simulink model "ORMComponent"  (R2024a)
settings: Solver=FixedStepAuto  StartTime=0.0  StopTime=10.0  RelTol=1e-3
settings Model: DataDictionary=untitled_dict1.sldd  Creator=diell  LastModifiedBy=diell
settings OptimizationCC: DefaultParameterBehavior=Inlined  EnhancedBackFolding=on  PassReuseOutputArgsAs=Individual arguments  ZeroExternalMemoryAtStartup=off  ZeroInternalMemoryAtStartup=off  OptimizeBlockOrder=speed  DifferentSizesBufferReuse=on  OptimizationCustomize=off  EfficientTunableParamExpr=on
settings DebuggingCC: ParameterTunabilityLossMsg=error
settings SFSimCC: MATLABDynamicMemAlloc=off
settings RTWCC: Description=Embedded Coder  SystemTargetFile=ert.tlc  TemplateMakefile=ert_default_tmf  TargetLang=C++
settings CodeAppCC: ForceParamTrailComments=on  IgnoreCustomStorageClasses=off  OperatorAnnotations=on  SimulinkDataObjDesc=on  SFDataObjDesc=on  InsertBlockDesc=on
settings ERTTargetCC: TargetLangStandard=C++11 (ISO)  GenerateSampleERTMain=on  CodeInterfacePackaging=C++ class  InlinedParameterPlacement=NonHierarchical  RootIOFormat=Structure reference  ERTCustomFileTemplate=example_file_process.tlc

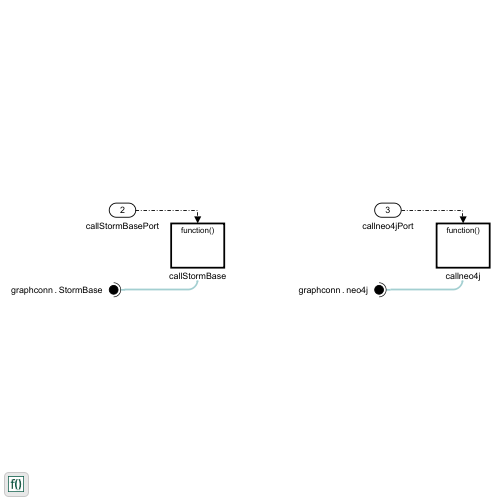
[thumbnail: Simulink's stored preview of the top-level diagram]
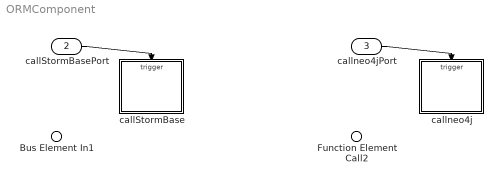
== system ORMComponent ==
  Function Element Call2 : Inport  AllowServiceAccess=on  PortName=graphconn  Element=neo4j
  Bus Element In1 : Inport  AllowServiceAccess=on  PortName=graphconn  Element=StormBase
  callStormBasePort : Inport  Port=2  OutputFunctionCall=on
  callneo4jPort : Inport  Port=3  OutputFunctionCall=on
  callStormBase : Subsystem
  callneo4j : Subsystem
  wires:
  callStormBasePort/1 -> callStormBase/Trigger
  callneo4jPort/1 -> callneo4j/Trigger

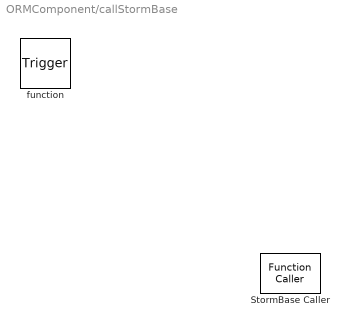
== system ORMComponent/callStormBase ==
  function : TriggerPort  TriggerType=function-call  VariantControl=(inherit)
  StormBase Caller : FunctionCaller  FunctionPrototype=orm = graphconn.StormBase(graphconn,path)  InputArgumentSpecifications=<Enter example>  OutputArgumentSpecifications=<Enter example>

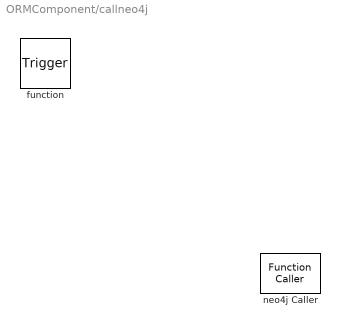
== system ORMComponent/callneo4j ==
  function : TriggerPort  TriggerType=function-call  VariantControl=(inherit)
  neo4j Caller : FunctionCaller  FunctionPrototype=graphconn = graphconn.neo4j(db,username,password)  InputArgumentSpecifications=<Enter example>  OutputArgumentSpecifications=<Enter example>
